simulink model "Base_FB"  (R2019b)
settings: Solver=VariableStepAuto  StartTime=0.0  StopTime=10.0  RelTol=1e-3
undefined symbols (not defined in the file): HIL, qc_get_step_size, sigbuilder_block, v_a_max
libraries: simulink_extras x7, quarc_library x4, cstblocks x3
settings Model: Creator=jesuc  LastModifiedBy=AleFire
settings DataIOCC: SaveFormat=Array  ReturnWorkspaceOutputs=off
settings DebuggingCC: SFMachineParentedDataDiag=error

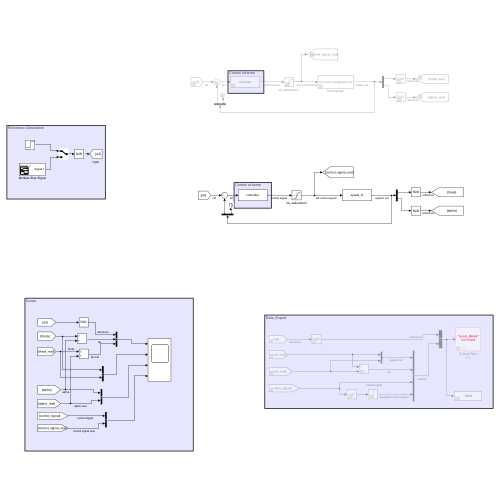
[thumbnail: Simulink's stored preview of the top-level diagram]
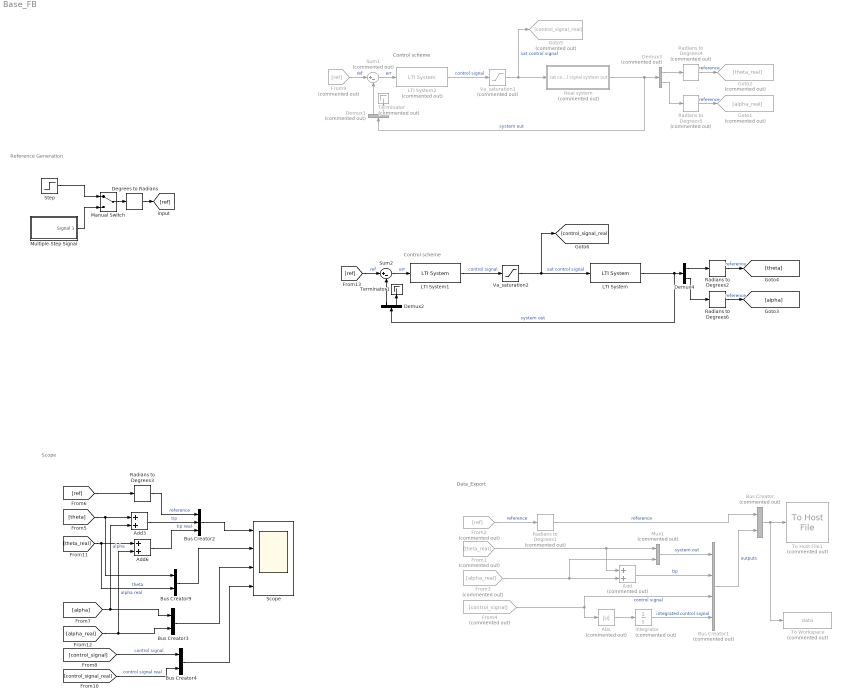
== system Base_FB ==
  note: Reference Generation
  note: Control scheme
  note: Scope
  note: Data_Export
  note: Control scheme
  Abs : Abs  Commented=on
  Add : Sum  Commented=on
  Add3 : Sum
  Add6 : Sum
  Bus Creator : BusCreator  Commented=on  Inputs=2
  Bus Creator1 : BusCreator  Commented=on  Inputs=4
  Bus Creator2 : BusCreator  Inputs=3
  Bus Creator3 : BusCreator  Inputs=2
  Bus Creator4 : BusCreator  Inputs=2
  Bus Creator9 : BusCreator  Inputs=2
  Degrees to Radians : simulink_extras/Transformations/Degrees to Radians
  Demux1 : Demux  Commented=on  Outputs=2
  Demux2 : Demux  Outputs=2
  Demux3 : Demux  Commented=on  Outputs=2
  Demux4 : Demux  Outputs=2
  From1 : From  Commented=on  GotoTag=theta_real
  From2 : From  Commented=on  GotoTag=ref
  From3 : From  Commented=on  GotoTag=alpha_real
  From4 : From  Commented=on  GotoTag=control_signal
  From9 : From  Commented=on  GotoTag=ref
  Goto1 : Goto  Commented=on  GotoTag=alpha_real
  Goto2 : Goto  Commented=on  GotoTag=theta_real
  Goto5 : Goto  Commented=on  GotoTag=control_signal_real
  Integrator : Integrator  Commented=on
  LTI System : cstblocks/LTI System  sys=sysest_ct  IC=[]
  LTI System1 : cstblocks/LTI System  sys=controller  IC=[]
  LTI System2 : cstblocks/LTI System  Commented=on  sys=controller  IC=[]
  Manual Switch : ManualSwitch
  Multiple-Step Signal : Subsystem  Tag=STV Subsys  LoadFcn=sigbuilder_block('load');  StartFcn=sigbuilder_block('start');  StopFcn=sigbuilder_block('stop');  ClipboardFcn=sigbuilder_block('clipboard');  mask(Sigbuilder block){tuvar=[0:10]}
      mask help: Simulink:masks:SigbuilderBlock_MD
      mask init:
      | if ~strcmp(get_param(bdroot(gcbh),'SimulationStatus'),'stopped') tuvar = sigbuilder_block('maskInit'); end
      settings: CopyFcn=sigbuilder_block('copy');  DeleteFcn=sigbuilder_block('delete');  ModelCloseFcn=sigbuilder_block('modelClose');  PreSaveFcn=sigbuilder_block('preSave');  PauseFcn=sigbuilder_block('pause');  ContinueFcn=sigbuilder_block('continue');  NameChangeFcn=sigbuilder_block('namechange');  OpenFcn=sigbuilder_block('open',[437.6 199.2 550.4 400 ]);  CloseFcn=sigbuilder_block('close');
      mask Display: plot(0, 0, 100, 100,[2, 2, 32, 32, 2], [68, 8, 8, 68, 68],[32, 2], [38, 38], [32, 19, 2],[53, 60, 44], [32, 17, 17, 2],[16, 16, 31, 31]);txt = getActiveGroup(gcbh);text(2, 100, txt,'verticalAlignment', 'top');
  Mux1 : Mux  Commented=on  Inputs=2
  Radians to Degrees1 : simulink_extras/Transformations/Radians to Degrees  Commented=on
  Radians to Degrees2 : simulink_extras/Transformations/Radians to Degrees
  Radians to Degrees3 : simulink_extras/Transformations/Radians to Degrees
  Radians to Degrees4 : simulink_extras/Transformations/Radians to Degrees  Commented=on
  Radians to Degrees5 : simulink_extras/Transformations/Radians to Degrees  Commented=on
  Radians to Degrees6 : simulink_extras/Transformations/Radians to Degrees
  Real system : Subsystem  Commented=on
  Scope : Scope  NumInputPorts=4
  Step : Step  After=45  SampleTime=0
  Sum1 : Sum  Commented=on  Inputs=|+-
  Sum2 : Sum  Inputs=|+-
  Terminator : Terminator  Commented=on
  Terminator1 : Terminator
  To Host File1 : quarc_library/Sinks/To Host/To Host File  Commented=on  file_name=Sine tests\Sine_24_in_theta_alpha.mat  variable_name=data  decimation=1  sample_time=-1  file_format=MAT-file v.4  options=No header or footer  append=off  final_file_name=Sine tests\Sine_24_in_theta_alpha.mat  bitrate=2000000
  To Workspace : ToWorkspace  Commented=on  VariableName=data  SaveFormat=Timeseries  SampleTime=-1
  Va_saturation1 : Saturate  Commented=on  UpperLimit=v_a_max  LowerLimit=-v_a_max
  Va_saturation2 : Saturate  UpperLimit=v_a_max  LowerLimit=-v_a_max
  wires:
  Multiple-Step Signal/1(Signal 1) -> Manual Switch/2
  Step/1 -> Manual Switch/1
  Manual Switch/1 -> Degrees to Radians/1
  Degrees to Radians/1 -> [ref]
  Va_saturation1/1 -> Goto5/1, Real system/1(sat control signal)  "sat control signal"
  Sum1/1 -> LTI System2/1  "err"
  From9/1 -> Sum1/1  "ref"
  LTI System2/1 -> Va_saturation1/1  "control signal"
  [control_signal_real] -> Bus Creator4/2  "control signal real"
  From4/1 -> Abs/1, Bus Creator1/3  "control signal"
  [theta_real] -> Bus Creator9/2, Add6/1  "theta"
  Bus Creator1/1 -> Bus Creator/2  "outputs"
  [alpha_real] -> Bus Creator3/2, Add6/2  "alpha real"
  Radians to Degrees3/1 -> Bus Creator2/1  "reference"
  Abs/1 -> Integrator/1
  [ref] -> Radians to Degrees3/1
  Bus Creator9/1 -> Scope/2
  Bus Creator2/1 -> Scope/1
  Add6/1 -> Bus Creator2/3  "tip real"
  From3/1 -> Add/2, Mux1/2
  [alpha] -> Bus Creator3/1, Add3/2  "alpha"
  Bus Creator/1 -> To Workspace/1, To Host File1/1
  [control_signal] -> Bus Creator4/1  "control signal"
  Bus Creator4/1 -> Scope/4
  [theta] -> Bus Creator9/1, Add3/1
  Bus Creator3/1 -> Scope/3
  Add3/1 -> Bus Creator2/2  "tip"
  Mux1/1 -> Bus Creator1/1  "system out"
  Integrator/1 -> Bus Creator1/4  "integrated control signal"
  From2/1 -> Radians to Degrees1/1  "reference"
  From1/1 -> Add/1, Mux1/1
  Radians to Degrees1/1 -> Bus Creator/1  "reference"
  Add/1 -> Bus Creator1/2  "tip"
  Demux1/1 -> Sum1/2
  Demux1/2 -> Terminator/1
  Radians to Degrees4/1 -> Goto2/1  "reference"
  Demux3/1 -> Radians to Degrees4/1
  Demux3/2 -> Radians to Degrees5/1
  Radians to Degrees5/1 -> Goto1/1  "reference"
  Real system/1(system out) -> Demux3/1, Demux1/1  "system out"
  Sum2/1 -> LTI System1/1  "err"
  [ref] -> Sum2/1  "ref"
  Radians to Degrees2/1 -> [theta]  "reference"
  LTI System1/1 -> Va_saturation2/1  "control signal"
  Demux4/1 -> Radians to Degrees2/1
  Radians to Degrees6/1 -> [alpha]  "reference"
  Va_saturation2/1 -> LTI System/1, [control_signal_real]  "sat control signal"
  Demux4/2 -> Radians to Degrees6/1
  Demux2/2 -> Terminator1/1
  Demux2/1 -> Sum2/2
  LTI System/1 -> Demux4/1, Demux2/1  "system out"

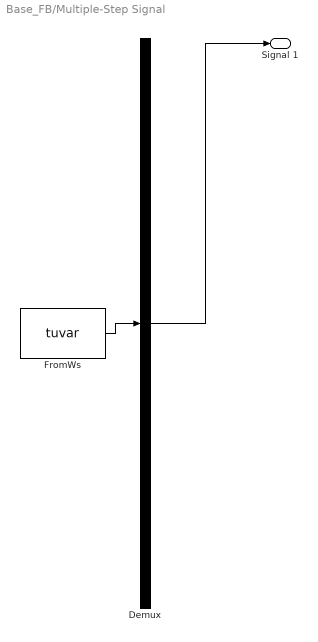
== system Base_FB/Multiple-Step Signal ==
  Demux : Demux  Tag=STV Demux  Outputs=1
      settings: DisplayOption=none
  FromWs : FromWorkspace  Tag=STV FromWs  VariableName=tuvar
      SigBuilderData=|
      | common.afterFinalStr = 'Extrapolate'
      | common.sampleTime = 0
      | dataSet.timeRange = [0 10]
      | dataSet.name = 'Group 1'
      | sbobj.Groups.Name = 'Group 1'
      | sbobj.Groups.Signals.Name = 'Signal 1'
      | sbobj.Groups.Signals.XData = [0 1 1 3 3 5 5 7 7 8.5 8.5 10]
      | sbobj.Groups.Signals.YData = [0.005 0.005 40 40 15 15 -30 -30 0 0 23 23]
  Signal 1 : Outport  Tag=STV Outport
  wires:
  Demux/1 -> Signal 1/1
  FromWs/1 -> Demux/1

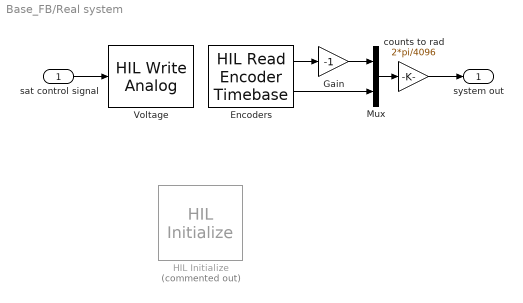
== system Base_FB/Real system ==
  sat control signal : Inport
  Encoders : quarc_library/Data Acquisition/Generic/Timebases/HIL Read Encoder Timebase  object_name=HIL-1  clock=0  channels=[0:1]  samples_in_buffer=max(ceil(1/qc_get_step_size), 1)  active=on  vector_output=off  data_type_mode=Inherit via back propagation  data_type=double
  Gain : Gain  Gain=-1
  HIL Initialize : quarc_library/Data Acquisition/Generic/Configuration/HIL Initialize  Priority=-99  Commented=on  object_name=HIL-1  board_type=q2_usb  board_number=0  board_options=d0=digital;d1=digital;led=auto;update_rate=normal;decimation=1  exclusive=off  active=off  hardware_clocks=[0]  clock_modes=[]  initial_clock_frequencies=[]  set_clock_params_at_start=off  set_clock_params_at_switch_in=off  set_clock_frequencies_at_start=off  set_clock_frequencies_at_switch_in=off  analog_input_channels=[0:1]  analog_input_configurations=[]  analog_input_maximums=10  analog_input_minimums=-10  set_analog_input_params_at_start=on  set_analog_input_params_at_switch_in=off  analog_output_channels=[0:1]  analog_output_maximums=10  analog_output_minimums=-10  initial_analog_outputs=[0]  final_analog_outputs=[0]  watchdog_analog_outputs=0  set_analog_output_params_at_start=on  set_analog_output_params_at_switch_in=off  set_analog_outputs_at_start=on  set_analog_outputs_at_switch_in=off  set_analog_outputs_at_terminate=on  set_analog_outputs_at_switch_out=off  set_analog_outputs_on_watchdog=off  digital_input_channels=[]  digital_output_channels=[]  digital_output_configuration=[]  initial_digital_outputs=[1]  final_digital_outputs=[1]  watchdog_digital_outputs=[1]  set_digital_output_params_at_start=off  set_digital_output_params_at_switch_in=off  set_digital_outputs_at_start=on  set_digital_outputs_at_switch_in=off  set_digital_outputs_at_terminate=on  set_digital_outputs_at_switch_out=off  set_digital_outputs_on_watchdog=off  encoder_channels=[0:1]  quadrature=[4]  encoder_filter_frequency=[]  initial_encoder_counts=[0]  set_encoder_params_at_start=on  set_encoder_params_at_switch_in=off  set_encoder_counts_at_start=on  set_encoder_counts_at_switch_in=off  pwm_channels=[]  pwm_modes=[0]  pwm_frequency=1/0.020  pwm_configuration=[]  pwm_alignment=[]  pwm_polarity=[]  pwm_leading_deadband=[]  pwm_trailing_deadband=[]  initial_pwm_outputs=[0]  final_pwm_outputs=[0]  watchdog_pwm_outputs=[0]  set_pwm_params_at_start=on  set_pwm_params_at_switch_in=off  set_pwm_outputs_at_start=on  set_pwm_outputs_at_switch_in=off  set_pwm_outputs_at_terminate=on  set_pwm_outputs_at_switch_out=off  set_pwm_outputs_on_watchdog=off  other_output_channels=[]  initial_other_outputs=[]  final_other_outputs=[]  watchdog_other_outputs=[]  set_other_outputs_at_start=off  set_other_outputs_at_switch_in=off  set_other_outputs_at_terminate=off  set_other_outputs_at_switch_out=off  set_other_outputs_on_watchdog=off
  Mux : Mux  Inputs=2
  Voltage : quarc_library/Data Acquisition/Generic/Immediate I//O/HIL Write Analog  object_name=HIL-1  channels=0  sample_time=-1  active=off  vector_input=off
  counts to rad : Gain  Gain=2*pi/4096
  system out : Outport
  wires:
  sat control signal/1 -> Voltage/1
  Encoders/1 -> Gain/1
  Encoders/2 -> Mux/2
  Mux/1 -> counts to rad/1
  Gain/1 -> Mux/1
  counts to rad/1 -> system out/1
